simulink model "bb_pid_rc_sl"  (Simulink 7.9)
settings: Solver=FixedStepDiscrete  StartTime=0.0  StopTime=inf  FixedStep=ts  RelTol=1e-3
values from neighbouring files (symbols this model uses):
  K_theta_rc = (pi/180)*(1.5/11.5)    (= 0.00227651641564)    [bb_pid_rc.m]
  kd = -(p1+p2+p3)/K_b    [bb_pid_hg.m]    (also in bb_pid_rc.m)
  kff = ki/alpha    [bb_pid_hg.m]    (also in bb_pid_rc.m)
  ki = -p1*p2*p3/K_b    [bb_pid_hg.m]    (also in bb_pid_rc.m)
  kp = (p1*p2 + p2*p3 + p3*p1)/K_b    [bb_pid_hg.m]    (also in bb_pid_rc.m)
  r1 = 20    [bb_lqr_hg.m]    (also in bb_lqr_servo_hg.m = 15; bb_pid_hg.m = 15; bb_pid_rc.m = 15)
  r2 = 20    [bb_lqr_hg.m]    (also in bb_lqr_servo_hg.m = 25; bb_pid_hg.m = 25; bb_pid_rc.m = 25)
  ts = 0.02    [sim_param.mat]
undefined symbols (not defined in the file or in its folder): denbd, denlpf, DiscIntNeverNeededParam, numbd, numlpf
libraries: arduino_io_lib x4, simulink x3
settings Model: Creator=hirata  LastModifiedBy=hirata
settings DebuggingCC: FcnCallInpInsideContextMsg=Use local settings
settings GRTTargetCC: CombineOutputUpdateFcns=off  GRTInterface=on

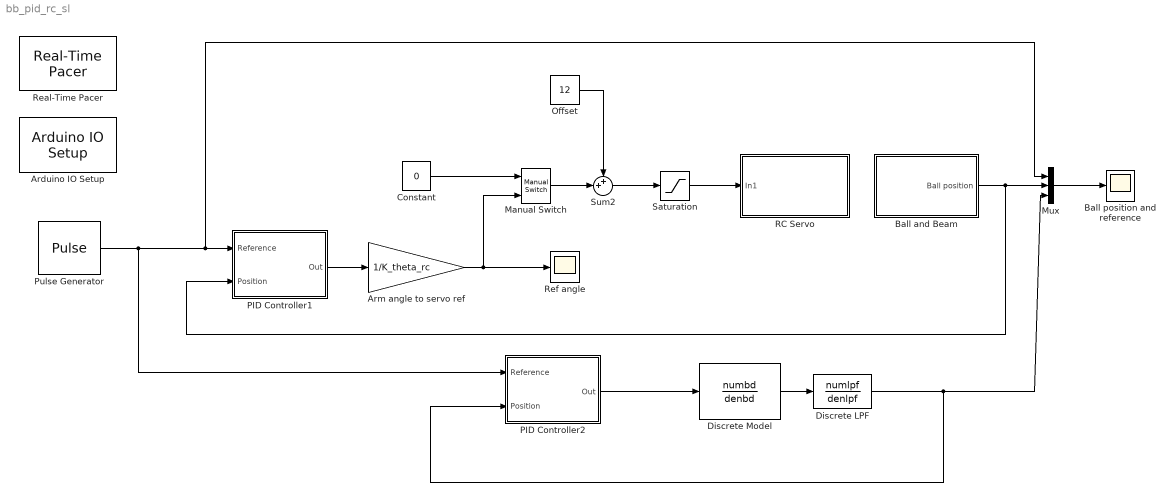
== system bb_pid_rc_sl ==
  Arduino IO Setup : arduino_io_lib/Arduino IO Setup  Priority=3  arduinoVar=Temporary arduino variable: Arduino1  workspaceVarName=a  comPort=COM3
  Arm angle to servo ref : Gain  Gain=1/K_theta_rc
  Ball and Beam : Subsystem
  Ball position and reference : Scope
      settings: TimeRange=30  YMin=-15  YMax=25
  Constant : Constant  Value=0
  Discrete LPF : DiscreteTransferFcn  Numerator=numlpf  Denominator=denlpf
  Discrete Model : DiscreteTransferFcn  Numerator=numbd  Denominator=denbd
  Manual Switch : simulink/Signal Routing/Manual Switch  sw=1  action=0  varsize=off
  Mux : Mux  Inputs=3
  Offset : Constant  Value=12  SampleTime=ts
  PID Controller1 : Subsystem
  PID Controller2 : Subsystem
  Pulse Generator : DiscretePulseGenerator  PulseType=Time based  Amplitude=r2-r1  Period=30  PulseWidth=50  PhaseDelay=10
  RC Servo : Subsystem
  Real-Time Pacer : arduino_io_lib/Real-Time Pacer  simTimePerRealTime=1
  Ref angle : Scope
      settings: TimeRange=30  YMin=-40  YMax=40  SaveName=ScopeData5
  Saturation : Saturate  UpperLimit=45  LowerLimit=-45
  Sum2 : Sum  Inputs=++|
  wires:
  Constant/1 -> Manual Switch/1
  Offset/1 -> Sum2/1
  Arm angle to servo ref/1 -> Manual Switch/2, Ref angle/1
  Sum2/1 -> Saturation/1
  Mux/1 -> Ball position and reference/1
  Manual Switch/1 -> Sum2/2
  Saturation/1 -> RC Servo/1(In1)
  Ball and Beam/1(Ball position) -> Mux/2, PID Controller1/2(Position)
  Pulse Generator/1 -> Mux/1, PID Controller1/1(Reference), PID Controller2/1(Reference)
  Discrete Model/1 -> Discrete LPF/1
  PID Controller2/1(Out) -> Discrete Model/1
  PID Controller1/1(Out) -> Arm angle to servo ref/1
  Discrete LPF/1 -> Mux/3, PID Controller2/2(Position)

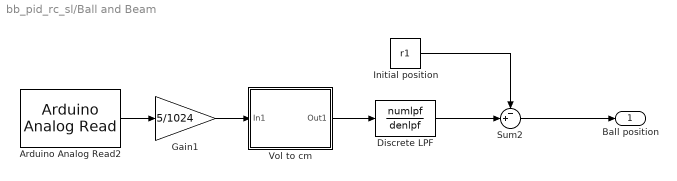
== system bb_pid_rc_sl/Ball and Beam ==
  Arduino Analog Read2 : arduino_io_lib/Arduino Analog Read  arduinoVar=Temporary arduino variable: Arduino1  arduinoPin=2  T=ts
  Discrete LPF : DiscreteTransferFcn  Numerator=numlpf  Denominator=denlpf
  Gain1 : Gain  Gain=5/1024
  Initial position : Constant  Value=r1
  Sum2 : Sum  Inputs=-+|
  Vol to cm : Subsystem
  Ball position : Outport
  wires:
  Arduino Analog Read2/1 -> Gain1/1
  Gain1/1 -> Vol to cm/1(In1)
  Vol to cm/1(Out1) -> Discrete LPF/1
  Initial position/1 -> Sum2/1
  Discrete LPF/1 -> Sum2/2
  Sum2/1 -> Ball position/1

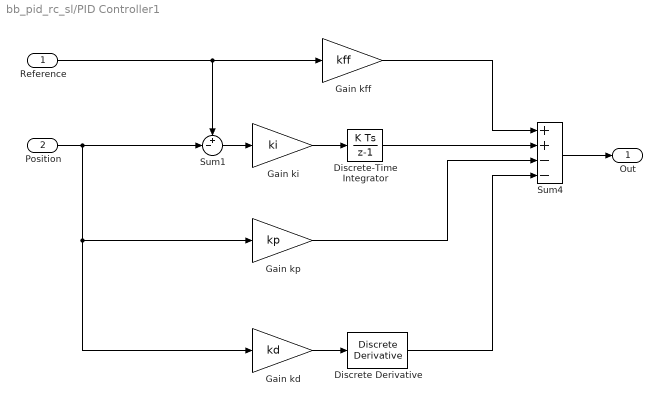
== system bb_pid_rc_sl/PID Controller1 ==
  Reference : Inport
  Position : Inport  Port=2
  Discrete Derivative : simulink/Discrete/Discrete Derivative  gainval=1.0  ICPrevScaledInput=0.0  InputProcessing=Inherited  OutMin=[]  OutMax=[]  OutDataType=fixdt(1, 16)  OutScaling=2^-10  DoSatur=off
  Discrete-Time Integrator : DiscreteIntegrator  SampleTime=ts  ICPrevOutput=DiscIntNeverNeededParam  ICPrevScaledInput=DiscIntNeverNeededParam
  Gain kd : Gain  Gain=kd
  Gain kff : Gain  Gain=kff
  Gain ki : Gain  Gain=ki
  Gain kp : Gain  Gain=kp
  Sum1 : Sum  Inputs=+-|
  Sum4 : Sum  Inputs=++--
  Out : Outport
  wires:
  Discrete Derivative/1 -> Sum4/4
  Gain kd/1 -> Discrete Derivative/1
  Gain kp/1 -> Sum4/3
  Gain kff/1 -> Sum4/1
  Sum4/1 -> Out/1
  Gain ki/1 -> Discrete-Time Integrator/1
  Discrete-Time Integrator/1 -> Sum4/2
  Position/1 -> Gain kd/1, Gain kp/1, Sum1/2
  Sum1/1 -> Gain ki/1
  Reference/1 -> Gain kff/1, Sum1/1

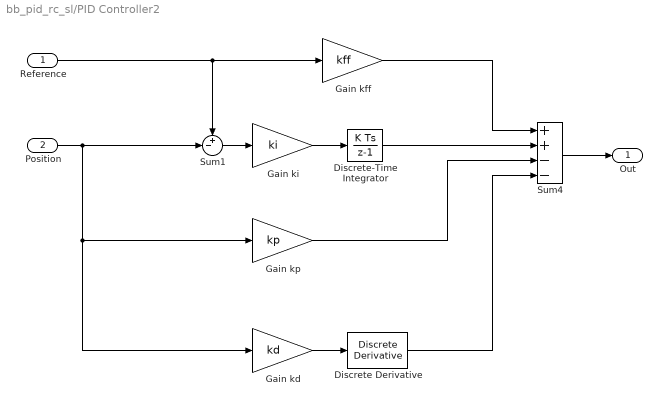
== system bb_pid_rc_sl/PID Controller2 ==
  Reference : Inport
  Position : Inport  Port=2
  Discrete Derivative : simulink/Discrete/Discrete Derivative  gainval=1.0  ICPrevScaledInput=0.0  InputProcessing=Inherited  OutMin=[]  OutMax=[]  OutDataType=fixdt(1, 16)  OutScaling=2^-10  DoSatur=off
  Discrete-Time Integrator : DiscreteIntegrator  SampleTime=ts  ICPrevOutput=DiscIntNeverNeededParam  ICPrevScaledInput=DiscIntNeverNeededParam
  Gain kd : Gain  Gain=kd
  Gain kff : Gain  Gain=kff
  Gain ki : Gain  Gain=ki
  Gain kp : Gain  Gain=kp
  Sum1 : Sum  Inputs=+-|
  Sum4 : Sum  Inputs=++--
  Out : Outport
  wires:
  Discrete Derivative/1 -> Sum4/4
  Gain kd/1 -> Discrete Derivative/1
  Gain kp/1 -> Sum4/3
  Gain kff/1 -> Sum4/1
  Sum4/1 -> Out/1
  Gain ki/1 -> Discrete-Time Integrator/1
  Discrete-Time Integrator/1 -> Sum4/2
  Position/1 -> Gain kd/1, Gain kp/1, Sum1/2
  Sum1/1 -> Gain ki/1
  Reference/1 -> Gain kff/1, Sum1/1

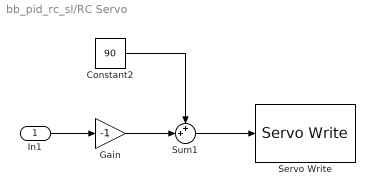
== system bb_pid_rc_sl/RC Servo ==
  In1 : Inport
  Constant2 : Constant  Value=90  SampleTime=ts
  Gain : Gain  Gain=-1
  Servo Write : arduino_io_lib/Servo Write  arduinoVar=Temporary arduino variable: Arduino1  pinNum=10  T=ts
  Sum1 : Sum  Inputs=++|
  wires:
  Sum1/1 -> Servo Write/1
  Constant2/1 -> Sum1/1
  In1/1 -> Gain/1
  Gain/1 -> Sum1/2

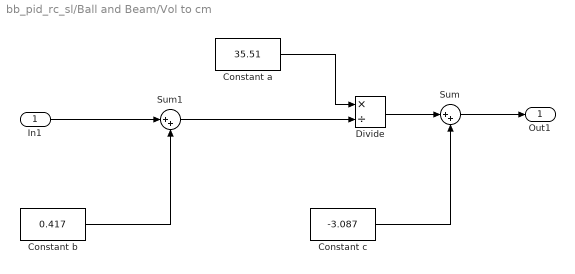
== system bb_pid_rc_sl/Ball and Beam/Vol to cm ==
  In1 : Inport
  Constant a : Constant  Value=35.51
  Constant b : Constant  Value=0.417
  Constant c : Constant  Value=-3.087
  Divide : Product  Inputs=*/
  Sum : Sum  Inputs=|++
  Sum1 : Sum  Inputs=|++
  Out1 : Outport
  wires:
  Constant b/1 -> Sum1/2
  Sum1/1 -> Divide/2
  In1/1 -> Sum1/1
  Constant c/1 -> Sum/2
  Sum/1 -> Out1/1
  Divide/1 -> Sum/1
  Constant a/1 -> Divide/1
